simulink model "EtudeDesDifferentSystemDePremierOrdre"  (R2017a)
settings: Solver=VariableStepAuto  StartTime=0.0  StopTime=100  RelTol=1e-3
values from neighbouring files (symbols this model uses):
  K1 = 1    [DeclarationdesVariables.m]
  K2 = 5    [DeclarationdesVariables.m]
  K3 = 10    [DeclarationdesVariables.m]
  T1 = 0.5    [DeclarationdesVariables.m]
  T2 = 2    [DeclarationdesVariables.m]
  T3 = 5    [DeclarationdesVariables.m]
settings Model: Creator=PC  LastModifiedBy=PC

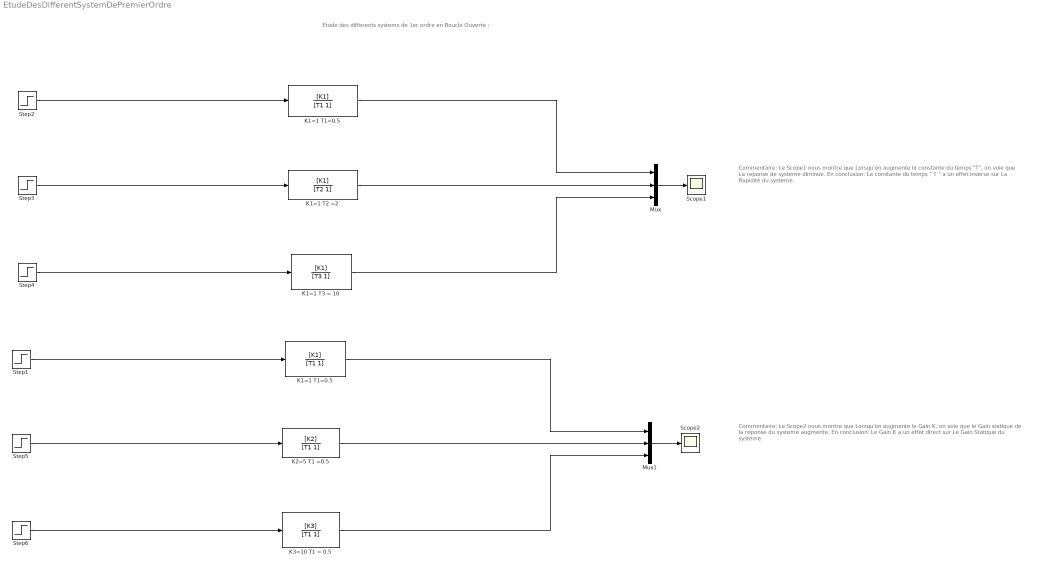
== system EtudeDesDifferentSystemDePremierOrdre ==
  note: Commentaire:
      | Le Scope2 nous montre que Lorsqu'on augmente le Gain K, on voie que le Gain statique de la reponse du systeme augmente.
      | En conclusion:
      | Le Gain K a un effet direct sur Le Gain Statique du systeme.
  note: Commentaire:
      | Le Scope1 nous montre que Lorsqu'on augmente la constante du temps "T", on voie que La reponse de systeme diminue.
      | En conclusion:
      | La constante du temps " T " a un effet inverse sur La Rapidité du systeme.
  note: Etude des differents systems de 1er ordre en Boucle Ouverte :
  K1=1 T1=0.5 : TransferFcn  Numerator=[K1]  Denominator=[T1 1]
  "K1=1 T1=0.5 " : TransferFcn  Numerator=[K1]  Denominator=[T1 1]
  "K1=1 T2 =2 " : TransferFcn  Numerator=[K1]  Denominator=[T2 1]
  "K1=1 T3 = 10 " : TransferFcn  Numerator=[K1]  Denominator=[T3 1]
  "K2=5 T1 =0.5 " : TransferFcn  Numerator=[K2]  Denominator=[T1 1]
  K3=10 T1 = 0.5 : TransferFcn  Numerator=[K3]  Denominator=[T1 1]
  Mux : Mux  Inputs=3
  Mux1 : Mux  Inputs=3
  "Scope1 " : Scope
  "Scope2 " : Scope
  Step{1..6} (6 alike) : Step  Time=0  SampleTime=0
  wires:
  Step4/1 -> "K1=1 T3 = 10 "/1
  Step3/1 -> "K1=1 T2 =2 "/1
  Step2/1 -> "K1=1 T1=0.5 "/1
  "K1=1 T1=0.5 "/1 -> Mux/1
  "K1=1 T2 =2 "/1 -> Mux/2
  "K1=1 T3 = 10 "/1 -> Mux/3
  Mux/1 -> "Scope1 "/1
  Mux1/1 -> "Scope2 "/1
  K3=10 T1 = 0.5/1 -> Mux1/3
  "K2=5 T1 =0.5 "/1 -> Mux1/2
  K1=1 T1=0.5/1 -> Mux1/1
  Step1/1 -> K1=1 T1=0.5/1
  Step5/1 -> "K2=5 T1 =0.5 "/1
  Step6/1 -> K3=10 T1 = 0.5/1
